simulink model "SOC_model_Code_Gen"  (R2026a)
settings: Solver=FixedStepDiscrete  StopTime=100  FixedStep=1
InitFcn:
  | clear
  | S = load("01_TEST_LGHG2@n10degC_Norm_(05_Inputs).mat");
  | steps = size(S.X,2);
  | t = (0:(steps-1))';
  | X_in = timeseries(single(S.X'), t);
  | true_SOC = timeseries(single(S.Y'), t);
libraries: deeplib x3
settings Model: SILPILModeSetting=veronly  LastModifiedBy=wenzheli
settings HardwareCC: ProdBitPerLong=64.0  ProdHWDeviceType=Intel->x86-64 (Linux 64)
settings SFSimCC: SimTargetLang=C++
settings RTWCC: SystemTargetFile=ert.tlc  PortableWordSizes=on  CodeExecutionProfiling=on  CodeProfilingSaveOptions=MetricsOnly  CodeProfilingInstrumentation=coarse  DataTypeReplacement=CDataTypesFixedWidth  Description=Embedded Coder
settings ERTTargetCC: MaxIdInt64=INT64_MAX  MinIdInt64=INT64_MIN  MaxIdUint64=UINT64_MAX  MaxIdInt32=INT32_MAX  MinIdInt32=INT32_MIN  MaxIdUint32=UINT32_MAX  MaxIdInt16=INT16_MAX  MinIdInt16=INT16_MIN  MaxIdUint16=UINT16_MAX  MaxIdInt8=INT8_MAX  MinIdInt8=INT8_MIN  MaxIdUint8=UINT8_MAX  GenerateSampleERTMain=on  SupportVariableSizeSignals=on

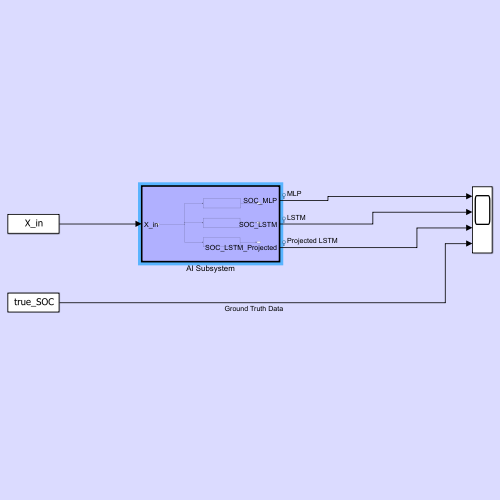
[thumbnail: Simulink's stored preview of the top-level diagram]
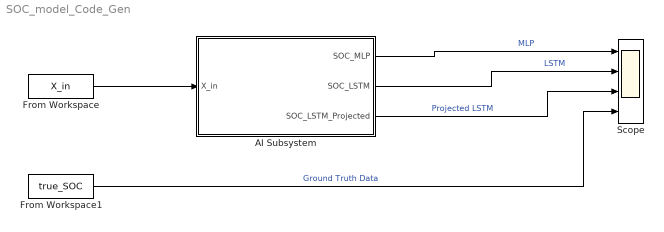
== system SOC_model_Code_Gen ==
  AI Subsystem : Subsystem  TreatAsAtomicUnit=on
      settings: RTWSystemCode=Nonreusable function
  From Workspace : FromWorkspace  VariableName=X_in  SampleTime=1
  From Workspace1 : FromWorkspace  VariableName=true_SOC  SampleTime=1
  Scope : Scope  NumInputPorts=4
      settings: ActiveDisplayYMinimum=-1.8850061940228491  ActiveDisplayYMaximum=2.2659924579613122
  wires:
  AI Subsystem/1(SOC_MLP) -> Scope/1  "MLP"
  AI Subsystem/3(SOC_LSTM_Projected) -> Scope/3  "Projected LSTM"
  AI Subsystem/2(SOC_LSTM) -> Scope/2  "LSTM"
  From Workspace/1 -> AI Subsystem/1(X_in)
  From Workspace1/1 -> Scope/4  "Ground Truth Data"

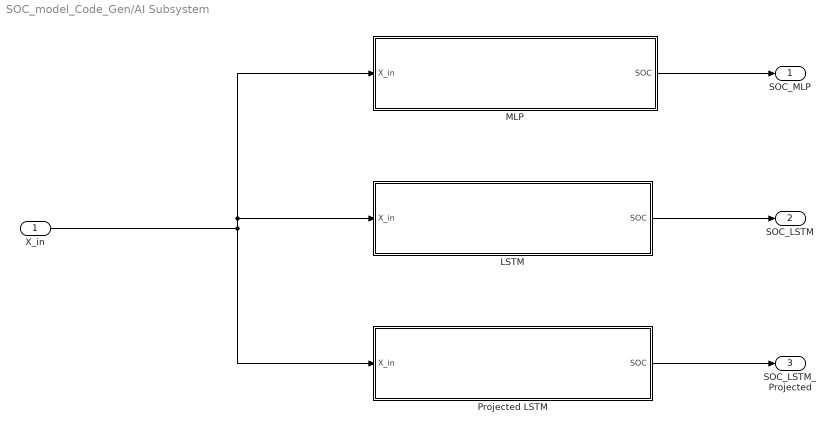
== system SOC_model_Code_Gen/AI Subsystem ==
  X_in : Inport
  LSTM : Subsystem  TreatAsAtomicUnit=on
      settings: RTWSystemCode=Nonreusable function
  MLP : Subsystem  TreatAsAtomicUnit=on
      settings: RTWSystemCode=Nonreusable function
  Projected LSTM : Subsystem  TreatAsAtomicUnit=on
      settings: RTWSystemCode=Nonreusable function
  SOC_MLP : Outport
  SOC_LSTM : Outport  Port=2
  SOC_LSTM_Projected : Outport  Port=3
  wires:
  Projected LSTM/1(SOC) -> SOC_LSTM_Projected/1
  LSTM/1(SOC) -> SOC_LSTM/1
  MLP/1(SOC) -> SOC_MLP/1
  X_in/1 -> MLP/1(X_in), LSTM/1(X_in), Projected LSTM/1(X_in)

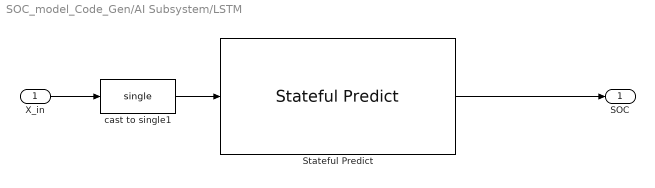
== system SOC_model_Code_Gen/AI Subsystem/LSTM ==
  X_in : Inport
  Stateful Predict : deeplib/Stateful Predict  Network=Network from MAT-file  NetworkFunction=untitled  NetworkFilePath=trainedNetwork.mat  SimulateUsing=Auto mode  InputDataFormats={ 'sequenceinput', 'CBT' }  SampleTime=-1  ForceInterpretedSim=off  EnableDLNetwork=on  LastKnownNetworkFilePath=''  LastKnownNetworkTimeStamp=''
  cast to single1 : DataTypeConversion  OutDataTypeStr=single  SaturateOnIntegerOverflow=off  RndMeth=Floor
  SOC : Outport
  wires:
  Stateful Predict/1 -> SOC/1
  X_in/1 -> cast to single1/1
  cast to single1/1 -> Stateful Predict/1

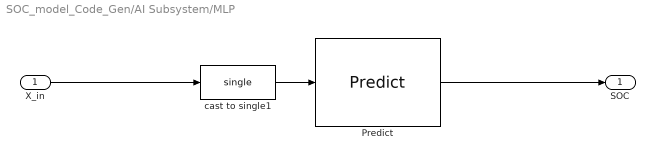
== system SOC_model_Code_Gen/AI Subsystem/MLP ==
  X_in : Inport
  Predict : deeplib/Predict  Network=Network from MAT-file  NetworkFunction=squeezenet  NetworkFilePath=netPyTorchMLP.mat  MiniBatchSize=128  SimulateUsing=Auto mode  InputDataFormats={'input_1', 'UU';}  Predictions=on  Activations={}  ForceInterpretedSim=off  EnableDLNetwork=on  LastKnownNetworkFilePath='netPyTorchMLP.mat'  LastKnownNetworkTimeStamp=740113.40938657405786216259002685546875
  cast to single1 : DataTypeConversion  OutDataTypeStr=single  SaturateOnIntegerOverflow=off  RndMeth=Floor
  SOC : Outport
  wires:
  Predict/1 -> SOC/1
  X_in/1 -> cast to single1/1
  cast to single1/1 -> Predict/1

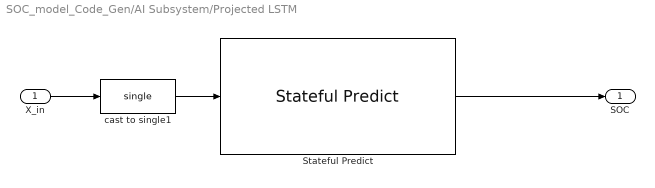
== system SOC_model_Code_Gen/AI Subsystem/Projected LSTM ==
  X_in : Inport
  Stateful Predict : deeplib/Stateful Predict  Network=Network from MAT-file  NetworkFunction=untitled  NetworkFilePath=dlnetFineTuned.mat  SimulateUsing=Auto mode  InputDataFormats={ 'sequenceinput', 'CBT' }  SampleTime=-1  ForceInterpretedSim=off  EnableDLNetwork=on  LastKnownNetworkFilePath=''  LastKnownNetworkTimeStamp=''
  cast to single1 : DataTypeConversion  OutDataTypeStr=single  SaturateOnIntegerOverflow=off  RndMeth=Floor
  SOC : Outport
  wires:
  Stateful Predict/1 -> SOC/1
  X_in/1 -> cast to single1/1
  cast to single1/1 -> Stateful Predict/1
